simulink model "PGA_MPC_MODEL"  (R2024b)
settings: Solver=ode4  StartTime=0.0  StopTime=180  FixedStep=0.0005  RelTol=1e-3
values from neighbouring files (symbols this model uses):
  Road_Curvature_Map = [Global_S, Global_K]    [Road_Condition_Info.m]
  Road_Mu_Map = [Global_S, Global_Mu]    [Road_Condition_Info.m]
  Target_Speed_Map = [Global_S, Global_Vx]    [Road_Condition_Info.m]
undefined symbols (not defined in the file or in its folder): MotorData, Sim_Mu_Set, Sim_Vx_Set
libraries: Solver_SF x1
(part 1 of 3)
settings Model: Creator=zlm22  LastModifiedBy=zlm22
settings SolverCC: InsertRTBMode=Always
settings RTWCC: BuildConfiguration=Faster Runs

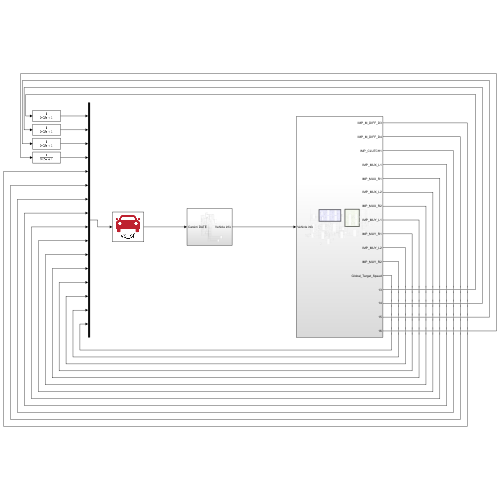
[thumbnail: Simulink's stored preview of the top-level diagram]
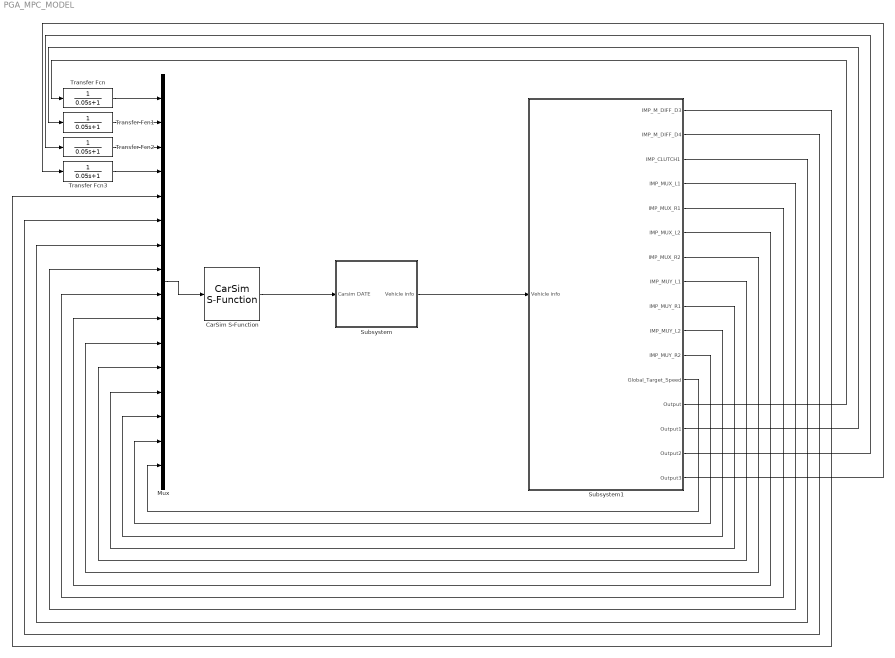
== system PGA_MPC_MODEL ==
  CarSim S-Function : Solver_SF/CarSim S-Function  Priority=1  SIMFILE=simfile.sim  Run_RTs=off  vs_state_ind=Run  StopMode_ind=Vehicle Model
  Mux : Mux  Inputs=16
  Subsystem : Subsystem
  Subsystem1 : Subsystem
  Transfer Fcn{,1..3} (4 alike) : TransferFcn  Denominator=[0.05 1]
  wires:
  Transfer Fcn/1 -> Mux/1
  Transfer Fcn1/1 -> Mux/2
  Transfer Fcn2/1 -> Mux/3
  Transfer Fcn3/1 -> Mux/4
  Subsystem/1(Vehicle info) -> Subsystem1/1(Vehicle info)
  Subsystem1/1(IMP_M_DIFF_D3) -> Mux/5
  Subsystem1/2(IMP_M_DIFF_D4) -> Mux/6
  Subsystem1/3(IMP_CLUTCH1) -> Mux/7
  Subsystem1/4(IMP_MUX_L1) -> Mux/8
  Subsystem1/5(IMP_MUX_R1) -> Mux/9
  Subsystem1/6(IMP_MUX_L2) -> Mux/10
  Subsystem1/7(IMP_MUX_R2) -> Mux/11
  Subsystem1/8(IMP_MUY_L1) -> Mux/12
  Subsystem1/9(IMP_MUY_R1) -> Mux/13
  Subsystem1/10(IMP_MUY_L2) -> Mux/14
  Subsystem1/11(IMP_MUY_R2) -> Mux/15
  Subsystem1/12(Global_Target_Speed) -> Mux/16
  Subsystem1/13(Output) -> Transfer Fcn/1
  Subsystem1/14(Output1) -> Transfer Fcn1/1
  Subsystem1/15(Output2) -> Transfer Fcn2/1
  Subsystem1/16(Output3) -> Transfer Fcn3/1
  Mux/1 -> CarSim S-Function/1
  CarSim S-Function/1 -> Subsystem/1(Carsim DATE)

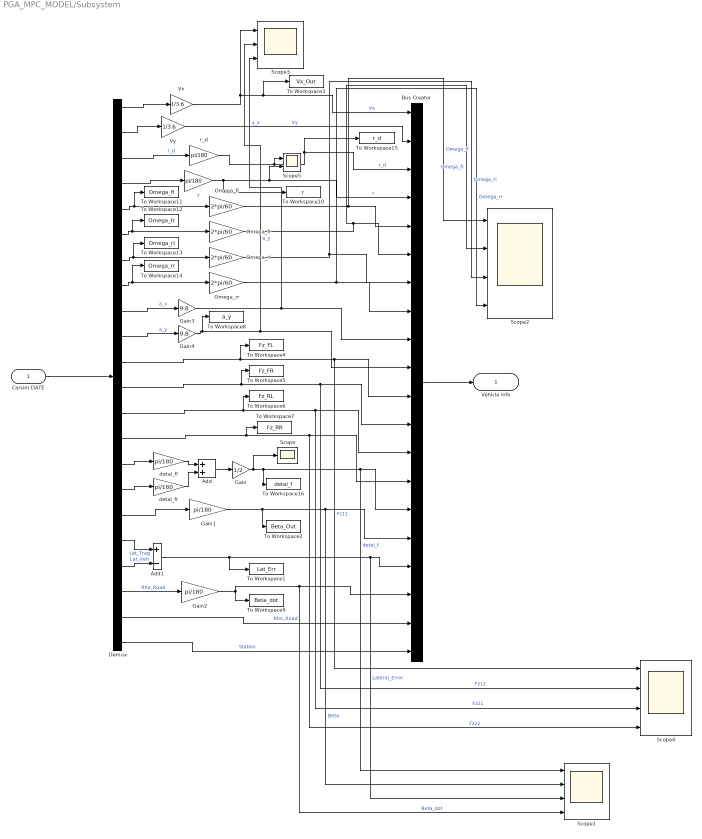
== system PGA_MPC_MODEL/Subsystem ==
  Carsim DATE : Inport
  Add : Sum
  Add1 : Sum  Inputs=+-
  Bus Creator : BusCreator  Inputs=20
  Demux : Demux  Outputs=22
  Gain : Gain  Gain=1/2
  Gain1 : Gain  Gain=pi/180
  Gain2 : Gain  Gain=pi/180
  Gain3 : Gain  Gain=9.8
  Gain4 : Gain  Gain=9.8
  Omega_fl : Gain  Gain=2*pi/60
  Omega_fr : Gain  Gain=2*pi/60
  Omega_rl : Gain  Gain=2*pi/60
  Omega_rr : Gain  Gain=2*pi/60
  Scope : Scope
  Scope1 : Scope  NumInputPorts=4
  Scope2 : Scope  NumInputPorts=4
  Scope3 : Scope  NumInputPorts=3
  Scope4 : Scope  NumInputPorts=4
  Scope5 : Scope  NumInputPorts=2
  To Workspace1 : ToWorkspace  VariableName=Lat_Err  SampleTime=-1
  To Workspace10 : ToWorkspace  VariableName=r  SampleTime=-1
  To Workspace11 : ToWorkspace  VariableName=Omega_fl  SampleTime=-1
  To Workspace12 : ToWorkspace  VariableName=Omega_fr  SampleTime=-1
  To Workspace13 : ToWorkspace  VariableName=Omega_rl  SampleTime=-1
  To Workspace14 : ToWorkspace  VariableName=Omega_rr  SampleTime=-1
  To Workspace15 : ToWorkspace  VariableName=r_d  SampleTime=-1
  To Workspace16 : ToWorkspace  VariableName=detal_f  SampleTime=-1
  To Workspace2 : ToWorkspace  VariableName=Beta_Out  SampleTime=-1
  To Workspace3 : ToWorkspace  VariableName=Vx_Out  SampleTime=-1
  To Workspace4 : ToWorkspace  VariableName=Fz_FL  SaveFormat=Timeseries  SampleTime=-1
  To Workspace5 : ToWorkspace  VariableName=Fz_FR  SaveFormat=Timeseries  SampleTime=-1
  To Workspace6 : ToWorkspace  VariableName=Fz_RL  SaveFormat=Timeseries  SampleTime=-1
  To Workspace7 : ToWorkspace  VariableName=Fz_RR  SaveFormat=Timeseries  SampleTime=-1
  To Workspace8 : ToWorkspace  VariableName=a_y  SampleTime=-1
  To Workspace9 : ToWorkspace  VariableName=Beta_dot  SampleTime=-1
  Vx : Gain  Gain=1/3.6
  Vy : Gain  Gain=1/3.6
  detal_fl : Gain  Gain=pi/180
  detal_fr : Gain  Gain=pi/180
  r : Gain  Gain=pi/180
  r_d : Gain  Gain=pi/180
  Vehicle info : Outport
  wires:
  Demux/3 -> r_d/1  "r_d"
  Demux/11 -> To Workspace4/1, Scope4/1, Bus Creator/11  "Fz11"
  Demux/8 -> To Workspace14/1, Omega_rr/1
  Vy/1 -> Bus Creator/2  "Vy"
  Demux/7 -> To Workspace13/1, Omega_rl/1
  Demux/14 -> To Workspace7/1, Scope4/4, Bus Creator/14  "Fz22"
  Demux/4 -> r/1
  Demux/5 -> To Workspace11/1, Omega_fl/1
  Demux/13 -> To Workspace6/1, Scope4/3, Bus Creator/13  "Fz21"
  Omega_rl/1 -> Scope2/3, Bus Creator/7  "Omega_rl"
  Demux/12 -> To Workspace5/1, Scope4/2, Bus Creator/12  "Fz12"
  Demux/16 -> detal_fr/1
  Omega_fr/1 -> Scope2/2, Bus Creator/6  "Omega_fr"
  Demux/6 -> To Workspace12/1, Omega_fr/1
  Demux/15 -> detal_fl/1
  Vx/1 -> Scope3/1, To Workspace3/1, Bus Creator/1  "Vx"
  r/1 -> Scope5/2, Bus Creator/4, To Workspace10/1  "r"
  Bus Creator/1 -> Vehicle info/1
  Omega_fl/1 -> Scope2/1, Bus Creator/5  "Omega_fl"
  Omega_rr/1 -> Scope2/4, Bus Creator/8  "Omega_rr"
  Demux/10 -> Gain4/1  "a_y"
  Demux/9 -> Gain3/1  "a_x"
  detal_fr/1 -> Add/2
  detal_fl/1 -> Add/1
  Add/1 -> Gain/1
  Gain/1 -> Scope/1, To Workspace16/1, Scope1/1, Bus Creator/15  "detal_f"
  Demux/1 -> Vx/1
  Demux/2 -> Vy/1
  Demux/17 -> Gain1/1
  Gain1/1 -> To Workspace2/1, Bus Creator/16, Scope1/2  "Beta"
  Gain2/1 -> Scope1/4, Bus Creator/18, To Workspace9/1  "Beta_dot"
  r_d/1 -> To Workspace15/1, Bus Creator/3, Scope5/1  "r_d"
  Carsim DATE/1 -> Demux/1
  Gain4/1 -> To Workspace8/1, Scope3/2, Bus Creator/10  "a_y"
  Gain3/1 -> Scope3/3, Bus Creator/9  "a_x"
  Demux/22 -> Bus Creator/20  "Station"
  Demux/21 -> Bus Creator/19  "Rho_Road"
  Demux/20 -> Gain2/1  "Rho_Road"
  Demux/18 -> Add1/1  "Lat_Trag"
  Demux/19 -> Add1/2  "Lat_Veh"
  Add1/1 -> To Workspace1/1, Scope1/3, Bus Creator/17  "Lateral_Error"

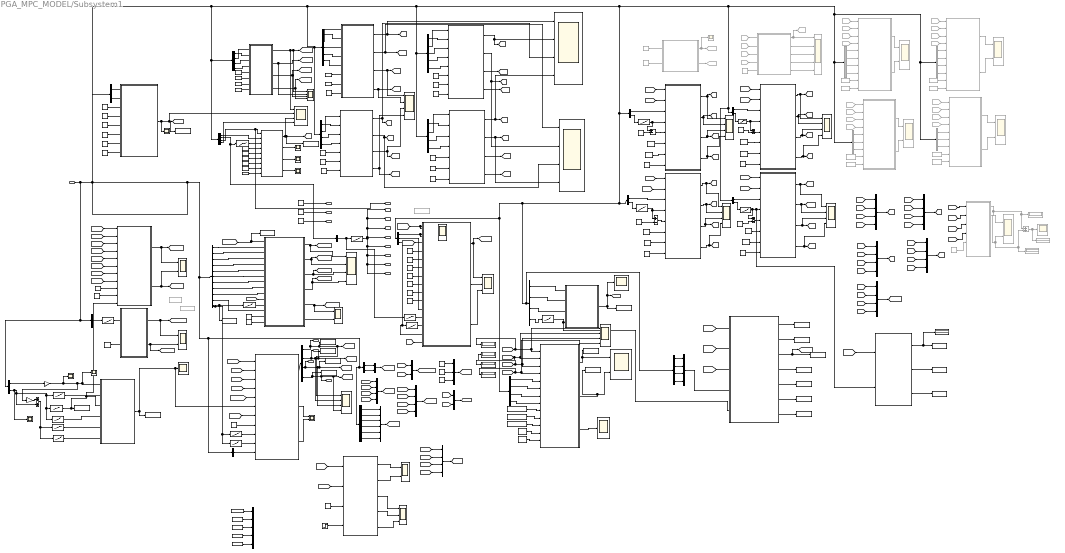
== system PGA_MPC_MODEL/Subsystem1 ==
  note: Subsystem3
  note: 轮胎力
  Vehicle info : Inport
  Add1 : Sum  Commented=on
  Add{2..4,6} (4 alike) : Sum  Inputs=+-
  Add5 : Sum
  Bus Creator : BusCreator  Inputs=6
  Bus Creator1 : BusCreator  Inputs=2
  Bus Selector : BusSelector  OutputSignals=Omega_fl,Omega_fr,Omega_rl,Omega_rr,Fz11,Fz12,Fz21,Fz22,a_y,Lateral_Error,Station
  Bus Selector1 : BusSelector  OutputSignals=Vx,detal_f,Fz11,Fz12,Fz21,Fz22
  Bus Selector10 : BusSelector  OutputSignals=Fz11,Station
  Bus Selector11 : BusSelector  OutputSignals=Fz21,Station
  Bus Selector12 : BusSelector  OutputSignals=Fz12,Station
  Bus Selector13 : BusSelector  OutputSignals=Fz22,Station
  Bus Selector15 : BusSelector  OutputSignals=Vx,Station
  Bus Selector16 : BusSelector  OutputSignals=detal_f
  Bus Selector17 : BusSelector  Commented=on  OutputSignals=Vx,Vy,r_d,detal_f
  Bus Selector18 : BusSelector  OutputSignals=Fz11,Fz12,Fz21,Fz22
  Bus Selector19 : BusSelector  Commented=on  OutputSignals=Vx,Vy,r_d,detal_f
  Bus Selector2 : BusSelector  OutputSignals=Beta,r_d
  Bus Selector20 : BusSelector  Commented=on  OutputSignals=Vx,Vy,r_d
  Bus Selector21 : BusSelector  Commented=on  OutputSignals=Vx,Vy,r_d
  Bus Selector22 : BusSelector  OutputSignals=Station
  Bus Selector23 : BusSelector  OutputSignals=detal_f,Station,Vx,r_d
  Bus Selector24 : BusSelector  OutputSignals=Station
  Bus Selector25 : BusSelector  OutputSignals=Omega_fl,Omega_fr,Omega_rl,Omega_rr
  Bus Selector26 : BusSelector  OutputSignals=Vx,detal_f,Beta
  Bus Selector27 : BusSelector  OutputSignals=Vx,Beta,Beta_dot,Station
  Bus Selector3 : BusSelector  OutputSignals=Vx,detal_f
  Bus Selector5 : BusSelector  OutputSignals=Vy,Vx,r_d,Omega_fl,detal_f
  Bus Selector6 : BusSelector  OutputSignals=Vy,Vx,r_d,detal_f
  Bus Selector7 : BusSelector  OutputSignals=Vy,Vx,r_d,Omega_fr,detal_f
  Bus Selector8 : BusSelector  OutputSignals=Vy,Vx,r_d,Omega_rl
  Bus Selector9 : BusSelector  OutputSignals=Vy,Vx,r_d,Omega_rr
  Constant{1,7,18,21,48} (5 alike) : Constant  Value=1.152
  Constant{2,8,10,13,49} (5 alike) : Constant  Value=1.528
  Constant{9,11,14,16..17,19} (6 alike) : Constant  Value=1.565
  Constant{12,15,20,22,54} (5 alike) : Constant  Value=0.347
  Constant{23..25,60,82} (5 alike) : Constant  Value=0
  Constant{26,73,81,84,91} (5 alike) : Constant  Value=0.05
  Constant27 : Constant  Commented=on  Value=3
  Constant28 : Constant  Commented=on  Value=0.001
  Constant{29,32,35,38} (4 alike) : Constant  Value=0.6
  Constant{3,31,37,50,79} (5 alike) : Constant  Value=63833
  Constant30 : Constant  Commented=on  Value=1.152
  Constant33 : Constant  Value=44230
  Constant{4,34,40,51,88} (5 alike) : Constant  Value=48729
  Constant36 : Constant  Value=57917
  Constant39 : Constant  Value=44230
  Constant41 : Constant  Commented=on  Value=0.347
  Constant{6,42,59,61,86} (5 alike) : Constant  Value=0.01
  Constant43 : Constant  Value=800
  Constant44 : Constant  Commented=on  Value=Sim_Mu_Set
  Constant45 : Constant  Value=MotorData.Speed_Axis
  Constant47 : Constant  Value=1810
  Constant5 : Constant  Value=1810
  Constant52 : Constant  Value=9.81
  Constant53 : Constant  Value=MotorData.Torque_Axis
  Constant55 : Constant  Value=1810
  Constant56 : Constant  Value=9.81
  Constant57 : Constant  Value=12
  Constant58 : Constant  Value=0.3
  Constant66 : Constant  Commented=on  Value=Sim_Vx_Set
  Constant68 : Constant  Commented=on  Value=Sim_Vx_Set
  Constant75 : Constant  Value=8000
  Constant76 : Constant  Value=12000
  Constant77 : Constant  Value=MotorData.Eff_Map
  Constant{78,92,94,96} (4 alike) : Constant  Commented=on  Value=1.565
  Constant80 : Constant  Value=0.005
  Constant83 : Constant  Value=18000
  Constant85 : Constant  Value=20000
  Constant87 : Constant  Value=15000  VectorParams1D=off
  Constant89 : Constant  Value=57917
  Constant90 : Constant  Commented=on  Value=1.152
  Constant93 : Constant  Commented=on  Value=1.528
  Constant95 : Constant  Commented=on  Value=1.528
  Constant97 : Constant  Commented=on  Value=0.01
  Demux : Demux
  Display{,1..3,8} (5 alike) : Display
  Display4 : Display  Commented=on
  Display5 : Display  Commented=on
  Display6 : Display  Commented=on
  From : From  Commented=on  GotoTag=Fx_fl
  From36 : From  Commented=on  GotoTag=Fx_fr
  From40 : From  Commented=on  GotoTag=Sx_fr
  From41 : From  Commented=on  GotoTag=Sy_fr
  From42 : From  Commented=on  GotoTag=Fy_rl
  From43 : From  Commented=on  GotoTag=Sx_rl
  From44 : From  Commented=on  GotoTag=Sy_rl
  From45 : From  Commented=on  GotoTag=Fx_rl
  From46 : From  Commented=on  GotoTag=Fy_rr
  From47 : From  Commented=on  GotoTag=Sx_rr
  From48 : From  Commented=on  GotoTag=Sy_rr
  From49 : From  Commented=on  GotoTag=Fx_rr
  From5 : From  Commented=on  GotoTag=Fy_fl
  From6 : From  Commented=on  GotoTag=Sx_fl
  From68 : From  Commented=on  GotoTag=Fx_fl
  From69 : From  Commented=on  GotoTag=Fx_fr
  From7 : From  Commented=on  GotoTag=Sy_fl
  From70 : From  Commented=on  GotoTag=Fx_rl
  From71 : From  Commented=on  GotoTag=Fx_rr
  From8 : From  Commented=on  GotoTag=Fx_fr
  Gain : Gain  Gain=3.6
  Gain2 : Gain  Gain=1.2
  Goto29 : Goto  Commented=on  GotoTag=mu_y
  Goto5 : Goto  Commented=on  GotoTag=mu_x
  MATLAB Function : MATLAB Function  TreatAsAtomicUnit=on  SystemSampleTime=0.01
  MATLAB Function1 : MATLAB Function  TreatAsAtomicUnit=on
  MATLAB Function10 : MATLAB Function  TreatAsAtomicUnit=on
  MATLAB Function12 : MATLAB Function  TreatAsAtomicUnit=on
  MATLAB Function14 : MATLAB Function  TreatAsAtomicUnit=on
  MATLAB Function15 : MATLAB Function  TreatAsAtomicUnit=on  SystemSampleTime=0.01
  MATLAB Function16 : MATLAB Function  Commented=on  TreatAsAtomicUnit=on
  MATLAB Function17 : MATLAB Function  TreatAsAtomicUnit=on
  MATLAB Function18 : MATLAB Function  TreatAsAtomicUnit=on
  MATLAB Function19 : MATLAB Function  TreatAsAtomicUnit=on  SystemSampleTime=0.01
  MATLAB Function2 : MATLAB Function  TreatAsAtomicUnit=on  SystemSampleTime=0.01
  MATLAB Function20 : MATLAB Function  Commented=on  TreatAsAtomicUnit=on
  MATLAB Function21 : MATLAB Function  Commented=on  TreatAsAtomicUnit=on  SystemSampleTime=0.01
  MATLAB Function22 : MATLAB Function  Commented=on  TreatAsAtomicUnit=on
  MATLAB Function23 : MATLAB Function  TreatAsAtomicUnit=on  SystemSampleTime=0.01
  MATLAB Function24 : MATLAB Function  Commented=on  TreatAsAtomicUnit=on
  MATLAB Function25 : MATLAB Function  Commented=on  TreatAsAtomicUnit=on
  MATLAB Function26 : MATLAB Function  TreatAsAtomicUnit=on
  MATLAB Function27 : MATLAB Function  TreatAsAtomicUnit=on
  MATLAB Function3 : MATLAB Function  TreatAsAtomicUnit=on  SystemSampleTime=0.01
  MATLAB Function4 : MATLAB Function  TreatAsAtomicUnit=on
  MATLAB Function5 : MATLAB Function  TreatAsAtomicUnit=on
  MATLAB Function6 : MATLAB Function  TreatAsAtomicUnit=on
  MATLAB Function7 : MATLAB Function  TreatAsAtomicUnit=on
  MATLAB Function8 : MATLAB Function  TreatAsAtomicUnit=on
  MATLAB Function9 : MATLAB Function  TreatAsAtomicUnit=on
  MU : Lookup_n-D  NumberOfTableDimensions=1  BreakpointsForDimension1=Road_Mu_Map(:, 1)  Table=Road_Mu_Map(:, 2)  InternalRulePriority=Speed  RndMeth=Simplest
  Mu{2..9,12..14} (11 alike) : Lookup_n-D  NumberOfTableDimensions=1  BreakpointsForDimension1=Road_Mu_Map(:, 1)  Table=Road_Mu_Map(:, 2)  InternalRulePriority=Speed  RndMeth=Simplest
  Mux : Mux  Inputs=2
  Mux{1,3,5..10,12} (9 alike) : Mux
  Mux13 : Mux  Inputs=5
  Mux2 : Mux  Inputs=2
  Mux4 : Mux  Inputs=3
  Radius{1..4} (4 alike) : Lookup_n-D  NumberOfTableDimensions=1  BreakpointsForDimension1=Road_Curvature_Map(:, 1)  Table=Road_Curvature_Map(:, 2)  InternalRulePriority=Speed  RndMeth=Simplest
  SI : Scope
  Scope{,1..2,5,27,37,45} (7 alike) : Scope  NumInputPorts=2
  Scope{10..14} (5 alike) : Scope  Commented=on  NumInputPorts=2
  Scope{3..4,6,9,15..18,20,28,30,48} (12 alike) : Scope  NumInputPorts=4
  Scope{8,19,21..22,32..34,44,49} (9 alike) : Scope
  Scope23 : Scope  Commented=on
  Scope24 : Scope  Commented=on  NumInputPorts=5
  Scope29 : Scope  NumInputPorts=3
  Scope47 : Scope  Commented=on
  Scope7 : Scope  NumInputPorts=3
  Step : Step  Time=0.01  Before=1  After=0  SampleTime=0.01
  T_max : Constant  Value=800
  T_min : Constant  Value=-200
  To Workspace : ToWorkspace  VariableName=SI_Out  SaveFormat=Timeseries  SampleTime=-1
  To Workspace10 : ToWorkspace  VariableName=R_ref  SampleTime=-1
  To Workspace12 : ToWorkspace  VariableName=beta_ref  SampleTime=-1
  To Workspace13 : ToWorkspace  VariableName=Sim_Station  SampleTime=-1
  To Workspace14 : ToWorkspace  VariableName=Mu  SampleTime=-1
  To Workspace17 : ToWorkspace  VariableName=Sx_abs_vec  SampleTime=-1
  To Workspace18 : ToWorkspace  VariableName=Sx_max  SampleTime=-1
  To Workspace19 : ToWorkspace  VariableName=Sx_rms  SampleTime=-1
  To Workspace2 : ToWorkspace  VariableName=NN_Weights  SampleTime=-1
  To Workspace20 : ToWorkspace  VariableName=Eta_vec  SampleTime=-1
  To Workspace21 : ToWorkspace  VariableName=Eta_max  SampleTime=-1
  To Workspace22 : ToWorkspace  VariableName=Eta_rms  SampleTime=-1
  To Workspace23 : ToWorkspace  VariableName=Slip_Debug_Info  SampleTime=-1
  To Workspace24 : ToWorkspace  VariableName=I_Sx  SampleTime=-1
  To Workspace25 : ToWorkspace  VariableName=I_Sx_norm  SampleTime=-1
  To Workspace26 : ToWorkspace  VariableName=I_Debug  SampleTime=-1
  To Workspace3 : ToWorkspace  VariableName=Total_Power_Out  SampleTime=-1
  To Workspace4 : ToWorkspace  VariableName=Motor_Torque_FL  SampleTime=-1
  To Workspace5 : ToWorkspace  VariableName=Motor_Torque_FR  SampleTime=-1
  To Workspace6 : ToWorkspace  VariableName=Motor_Torque_RL  SampleTime=-1
  To Workspace7 : ToWorkspace  VariableName=Motor_Torque_RR  SampleTime=-1
  To Workspace8 : ToWorkspace  VariableName=E_total_kWh  SampleTime=-1
  To Workspace9 : ToWorkspace  VariableName=P_total_kW  SampleTime=-1
  Vx1 : Lookup_n-D  NumberOfTableDimensions=1  BreakpointsForDimension1=Target_Speed_Map(:, 1)  Table=Target_Speed_Map(:, 2)  InternalRulePriority=Speed  RndMeth=Simplest
  Vx2 : Lookup_n-D  NumberOfTableDimensions=1  BreakpointsForDimension1=Target_Speed_Map(:, 1)  Table=Target_Speed_Map(:, 2)  InternalRulePriority=Speed  RndMeth=Simplest
  delta_T_max : Constant  Value=600
  unitire轮胎力 : MATLAB Function  TreatAsAtomicUnit=on
  侧偏角计算 : MATLAB Function  TreatAsAtomicUnit=on
  总需求扭矩 : Goto  Commented=on  GotoTag=Td
  横纵向附着系数 : MATLAB Function  Commented=on  TreatAsAtomicUnit=on
  IMP_M_DIFF_D3 : Outport
  IMP_M_DIFF_D4 : Outport  Port=2
  IMP_CLUTCH1 : Outport  Port=3
  IMP_MUX_L1 : Outport  Port=4
  IMP_MUX_R1 : Outport  Port=5
  IMP_MUX_L2 : Outport  Port=6
  IMP_MUX_R2 : Outport  Port=7
  IMP_MUY_L1 : Outport  Port=8
  IMP_MUY_R1 : Outport  Port=9
  IMP_MUY_L2 : Outport  Port=10
  IMP_MUY_R2 : Outport  Port=11
  Global_Target_Speed : Outport  Port=12
  Output : Outport  Port=13
  Output1 : Outport  Port=14
  Output2 : Outport  Port=15
  Output3 : Outport  Port=16
  wires:
  MATLAB Function5/1(Sx_fr) -> [Sx_fr], Scope9/2
  Bus Selector7/1 -> MATLAB Function5/2(Vy)  "<Vy>"
  Constant13/1 -> MATLAB Function7/5(lr)
  Constant21/1 -> MATLAB Function5/6(lf)
  MATLAB Function8/3(Fbar_x_rl) -> Scope17/3, [Fsx_rl]
  MATLAB Function6/1(Sx_rl) -> [Sx_rl], Scope9/3
  Constant14/1 -> MATLAB Function7/6(twr)
  MATLAB Function7/1(Sx_rr) -> [Sx_rr], Scope9/4
  Constant1/1 -> MATLAB Function4/3(lf)
  Bus Selector11/1 -> MATLAB Function8/3(Fz_rl)  "<Fz21>"
  MATLAB Function9/2(Fy_fr) -> Scope15/2, [Fy_fr]
  Bus Selector6/4 -> 侧偏角计算/4(delta_f_rad)  "<detal_f>"
  MATLAB Function5/2(Sy_fr) -> [Sy_fr], Scope28/2
  Constant47/1 -> MATLAB Function17/4(m)
  Bus Selector5/5 -> unitire轮胎力/5(delta_f)  "<detal_f>"
  [Sx_fr] -> MATLAB Function9/1(Sx_fr)
  Constant52/1 -> MATLAB Function17/9(g)
  MATLAB Function17/1(r_d) -> [r_ref], To Workspace10/1, Scope30/3  "r_ref"
  Constant15/1 -> MATLAB Function7/7(Re)
  MATLAB Function9/1(Fx_fr) -> Scope15/1, [Fx_fr]
  MATLAB Function10/1(Fx_rr) -> Scope18/1, [Fx_rr]
  MATLAB Function1/1(Fx_fl) -> [Fx_fl], Scope48/1
  MATLAB Function7/2(Sy_rr) -> Scope28/4, [Sy_rr]
  Constant2/1 -> MATLAB Function4/4(lr)
  MATLAB Function20/1(Td) -> Scope24/1, 总需求扭矩/1
  Constant38/1 -> MATLAB Function10/8(E)
  [Sy_fr] -> MATLAB Function9/2(Sy_fr)
  Constant9/1 -> 侧偏角计算/7(twf)
  Bus Selector10/1 -> MATLAB Function1/3(Fz_fl)  "<Fz11>"
  Bus Selector7/4 -> MATLAB Function5/4(omega_fr)  "<Omega_fr>"
  Constant4/1 -> MATLAB Function4/6(Kyr)
  Constant5/1 -> MATLAB Function4/7(m)
  Constant8/1 -> 侧偏角计算/6(lr)
  Constant27/1 -> 横纵向附着系数/1(road_condition)
  Bus Selector3/2 -> MATLAB Function4/2(delta_f)  "<detal_f>"
  Bus Selector3/1 -> MATLAB Function4/1(Vx)  "<Vx>"
  Constant6/1 -> MATLAB Function4/8(dt)
  Constant17/1 -> MATLAB Function5/7(twf)
  MATLAB Function4/1(beta_ref) -> Scope44/1, To Workspace12/1, [beta_ref], Scope30/2  "beta_ref"
  MATLAB Function1/3(Fbar_x_fl) -> Scope48/3, [Fsx_fl]
  Constant48/1 -> MATLAB Function17/5(lf)
  Constant3/1 -> MATLAB Function4/5(Kyf)
  MATLAB Function1/4(Fbar_y_fl) -> Scope48/4, [Fsy_fl]
  Constant29/1 -> MATLAB Function1/8(E)
  From68/1 -> MATLAB Function20/1(Fx_fl)
  Bus Selector8/4 -> MATLAB Function6/4(omega_rl)  "<Omega_rl>"
  MATLAB Function6/2(Sy_rl) -> Scope28/3, [Sy_rl]
  From71/1 -> MATLAB Function20/4(Fx_rr)
  Constant50/1 -> MATLAB Function17/7(Kf0)
  Bus Selector5/4 -> unitire轮胎力/4(omega_fl)  "<Omega_fl>"
  Bus Selector6/1 -> 侧偏角计算/2(Vy)  "<Vy>"
  Constant49/1 -> MATLAB Function17/6(lr)
  MATLAB Function8/4(Fbar_y_rl) -> Scope17/4, [Fsy_rl]
  MATLAB Function9/4(Fbar_y_fr) -> Scope15/4, [Fsy_fr]
  Constant51/1 -> MATLAB Function17/8(Kr0)
  MATLAB Function17/4(r_limit) -> Scope34/1
  MATLAB Function17/2(K_s) -> Scope32/1
  MATLAB Function17/3(r_ideal) -> Scope33/1
  Constant22/1 -> MATLAB Function5/8(Re)
  横纵向附着系数/1(mu_x) -> Scope47/1, Goto5/1
  Bus Selector12/1 -> MATLAB Function9/3(Fz_fr)  "<Fz12>"
  [Sx_fl] -> MATLAB Function1/1(Sx_fl)
  Bus Selector9/4 -> MATLAB Function7/4(omega_rr)  "<Omega_rr>"
  unitire轮胎力/1(Sx_fl) -> Scope9/1, [Sx_fl]
  From69/1 -> MATLAB Function20/2(Fx_fr)
  From70/1 -> MATLAB Function20/3(Fx_rl)
  Constant10/1 -> MATLAB Function6/5(lr)
  [Sy_rr] -> MATLAB Function10/2(Sy_rr)
  Constant41/1 -> MATLAB Function20/5(r_e)
  Constant35/1 -> MATLAB Function9/8(E)
  [Sy_rl] -> MATLAB Function8/2(Sy_rl)
  Constant7/1 -> 侧偏角计算/5(lf)
  MATLAB Function9/3(Fbar_x_fr) -> Scope15/3, [Fsx_fr]
  Bus Selector13/1 -> MATLAB Function10/3(Fz_rr)  "<Fz22>"
  MATLAB Function1/2(Fy_fl) -> [Fy_fl], Scope48/2
  MATLAB Function10/4(Fbar_y_rr) -> Scope18/4, [Fsy_rr]
  MATLAB Function10/2(Fy_rr) -> Scope18/2, [Fy_rr]
  MATLAB Function10/3(Fbar_x_rr) -> Scope18/3, [Fsx_rr]
  Mu5/1 -> Add6/1, MATLAB Function1/4(mu_x)
  [Sx_rr] -> MATLAB Function10/1(Sx_rr)
  Constant32/1 -> MATLAB Function8/8(E)
  MATLAB Function8/1(Fx_rl) -> Scope17/1, [Fx_rl]
  MATLAB Function8/2(Fy_rl) -> Scope17/2, [Fy_rl]
  [Sy_fl] -> MATLAB Function1/2(Sy_fl)
  Constant19/1 -> unitire轮胎力/7(twf)
  [Sx_rl] -> MATLAB Function8/1(Sx_rl)
  横纵向附着系数/2(mu_y) -> Goto29/1
  Constant28/1 -> 横纵向附着系数/2(slip_ratio)
  Bus Selector9/1 -> MATLAB Function7/2(Vy)  "<Vy>"
  Constant18/1 -> unitire轮胎力/6(lf)
  unitire轮胎力/2(Sy_fl) -> Scope28/1, [Sy_fl]
  Constant16/1 -> 侧偏角计算/8(twr)
  Constant11/1 -> MATLAB Function6/6(twr)
  Bus Selector8/1 -> MATLAB Function6/2(Vy)  "<Vy>"
  Constant20/1 -> unitire轮胎力/8(Re)
  Bus Selector5/1 -> unitire轮胎力/2(Vy)  "<Vy>"
  Vehicle info/1 -> Bus Selector15/1, Bus Selector24/1, Bus Selector/1, Bus Selector1/1, Bus Selector2/1, Bus Selector16/1, Bus Selector23/1, Bus Selector6/1, Bus Selector9/1, Bus Selector7/1, Bus Selector10/1, Bus Selector18/1, Bus Selector27/1, Bus Selector25/1, Bus Selector26/1, Bus Selector11/1, Bus Selector21/1, Bus Selector19/1, Bus Selector20/1, Bus Selector17/1, Bus Selector13/1, Bus Selector12/1, Bus Selector8/1, Bus Selector5/1, Bus Selector3/1
  MATLAB Function20/5(T_rr) -> Scope24/5
  MATLAB Function20/4(T_rl) -> Scope24/4
  MATLAB Function20/3(T_fr) -> Scope24/3
  MATLAB Function20/2(T_fl) -> Scope24/2
  [T_ZY_RR] -> Display3/1, Scope6/4, MATLAB Function2/4(T_rr)
  [T_ZY_RL] -> Display2/1, Scope6/3, MATLAB Function2/3(T_rl)
  [T_ZY_FL] -> Display/1, Scope6/1, MATLAB Function2/1(T_fl)
  [T_ZY_FR] -> Display1/1, Scope6/2, MATLAB Function2/2(T_fr)
  Bus Selector25/1 -> MATLAB Function2/5(w_fl)  "<Omega_fl>"
  Bus Selector25/2 -> MATLAB Function2/6(w_fr)  "<Omega_fr>"
  Bus Selector25/3 -> MATLAB Function2/7(w_rl)  "<Omega_rl>"
  MATLAB Function2/3(P_avg_kW) -> Scope49/1
  Constant55/1 -> MATLAB Function15/4(m)
  Constant56/1 -> MATLAB Function15/5(g)
  MATLAB Function15/1(T_total) -> [T_total], Scope7/1
  MATLAB Function18/1(Vx_safe_cmd) -> Scope45/1, [Vx_safe_cmd]
  MATLAB Function18/2(Ax_cmd_final) -> Scope45/2, [Ax_cmd_final]
  [Vx_safe_cmd] -> Scope37/1, MATLAB Function15/1(Vx_cmd)
  [Ax_cmd_final] -> MATLAB Function15/3(Ax_cmd)
  MATLAB Function2/2(E_total_kWh) -> To Workspace8/1, Scope2/2
  MATLAB Function2/1(P_total_kW) -> To Workspace9/1, Scope2/1
  Constant73/1 -> MATLAB Function18/2(dt)
  Bus Selector27/3 -> MATLAB Function19/3(Beta_dot)  "<Beta_dot>"
  MATLAB Function19/1(SI_Out) -> SI/1, [SI], To Workspace/1  "SI_Out"
  [Fy_fl] -> MATLAB Function23/1(Fy_fl)
  [Fy_fr] -> MATLAB Function23/2(Fy_fr)
  [Fy_rl] -> MATLAB Function23/3(Fy_rl)
  [Fy_rr] -> MATLAB Function23/4(Fy_rr)
  [alpha_fl] -> MATLAB Function23/5(Alpha_fl)
  [alpha_fr] -> MATLAB Function23/6(Alpha_fr)
  [alpha_rl] -> MATLAB Function23/7(Alpha_rl)
  [alpha_rr] -> MATLAB Function23/8(Alpha_rr)
  Constant88/1 -> MATLAB Function23/10(Cr0)
  Constant79/1 -> MATLAB Function23/9(Cf0)
  MATLAB Function23/1(Cf_eq) -> Scope5/1, [Cf_eq]
  MATLAB Function23/2(Cr_eq) -> Scope5/2, [Cr_eq]
  Constant23/1 -> IMP_M_DIFF_D3/1
  Constant24/1 -> IMP_M_DIFF_D4/1
  Constant25/1 -> IMP_CLUTCH1/1
  Mu3/1 -> IMP_MUX_R2/1, IMP_MUX_L2/1, IMP_MUX_R1/1, IMP_MUX_L1/1, IMP_MUY_L1/1, IMP_MUY_R1/1, IMP_MUY_L2/1, IMP_MUY_R2/1
  Constant81/1 -> Add2/2
  Constant84/1 -> Add3/2
  Add4/1 -> MATLAB Function8/5(mu_y)
  Mu7/1 -> MATLAB Function8/4(mu_x), Add4/1
  Constant91/1 -> Add4/2
  [T_total] -> To Workspace3/1, MATLAB Function3/1(T_total_req)
  Bus Selector/8 -> MATLAB Function3/9(Fz_rr)  "<Fz22>"
  Bus Selector/7 -> MATLAB Function3/8(Fz_rl)  "<Fz21>"
  Bus Selector/6 -> MATLAB Function3/7(Fz_fr)  "<Fz12>"
  Bus Selector/5 -> MATLAB Function3/6(Fz_fl)  "<Fz11>"
  Bus Selector/4 -> MATLAB Function3/5(w_rr)  "<Omega_rr>"
  Bus Selector/3 -> MATLAB Function3/4(w_rl)  "<Omega_rl>"
  Bus Selector/2 -> MATLAB Function3/3(w_fr)  "<Omega_fr>"
  Bus Selector/1 -> MATLAB Function3/2(w_fl)  "<Omega_fl>"
  Constant43/1 -> MATLAB Function3/14(T_motor_max)
  MATLAB Function3/5(Mode_Out) -> Scope/1, [Mode_Signal]
  MATLAB Function3/1(T_ref_fl) -> [T_ref_fl], Scope4/1
  MATLAB Function3/2(T_ref_fr) -> Scope4/2, [T_ref_fr]
  MATLAB Function3/3(T_ref_rl) -> [T_ref_rl], Scope4/3
  MATLAB Function3/4(T_ref_rr) -> [T_ref_rr], Scope4/4
  Constant42/1 -> MATLAB Function3/15(dt)
  [beta_ref] -> Mux/1
  [r_ref] -> Mux/2
  [T_ref_fl] -> Mux1/1
  [T_ref_fr] -> Mux1/2
  [T_ref_rl] -> Mux1/3
  [T_ref_rr] -> Mux1/4
  Mux1/1 -> [T_ref_upper]
  [Cf_eq] -> Mux2/1
  [Cr_eq] -> Mux2/2
  Mux2/1 -> [Stiffness_Input]
  Bus Selector1/3 -> Bus Creator/3  "<Fz11>"
  Bus Selector1/4 -> Bus Creator/4  "<Fz12>"
  Bus Selector1/5 -> Bus Creator/5  "<Fz21>"
  Bus Selector1/6 -> Bus Creator/6  "<Fz22>"
  Bus Creator/1 -> [Vehicle_State]
  Bus Selector2/1 -> Bus Creator1/1  "<Beta>"
  Bus Selector2/2 -> Bus Creator1/2  "<r_d>"
  Bus Creator1/1 -> [x_curr]
  T_min/1 -> Mux4/1
  T_max/1 -> Mux4/2
  delta_T_max/1 -> Mux4/3
  Mux4/1 -> [Constraints]
  [x_curr] -> MATLAB Function/1(x_curr)
  [x_ref] -> MATLAB Function/2(x_ref)
  [T_ref_upper] -> MATLAB Function/3(T_ref_upper_in)
  [Vehicle_State] -> MATLAB Function/4(Vehicle_State)
  [Stiffness_Input] -> MATLAB Function/5(Stiffness_Input)
  [Constraints] -> MATLAB Function/7(Constraints)
  MATLAB Function/2(Solver_Status) -> Scope1/1
  MATLAB Function/3(Debug_Info) -> Scope1/2
  MATLAB Function/1(T_final_opt) -> Demux/1
  Demux/1 -> Output/1, To Workspace4/1, [T_ZY_FL], Scope3/1  "F11"
  Demux/2 -> Output1/1, To Workspace5/1, [T_ZY_FR], Scope3/2  "F12"
  Demux/3 -> Output2/1, To Workspace6/1, [T_ZY_RL], Scope3/3  "F21"
  Demux/4 -> To Workspace7/1, Output3/1, Scope3/4, [T_ZY_RR]  "F22"
  Constant54/1 -> MATLAB Function15/6(r_e)
  Constant60/1 -> MATLAB Function15/10(is_reset)
  Constant58/1 -> MATLAB Function15/8(Ki)
  Constant57/1 -> MATLAB Function15/7(Kp)
  Constant59/1 -> MATLAB Function15/9(dt)
  MATLAB Function15/2(T_ff) -> Scope7/2
  MATLAB Function15/3(T_fb) -> Scope7/3
  [alpha_fl] -> Mux5/1
  [alpha_fr] -> Mux5/2
  [alpha_rl] -> Mux5/3
  [alpha_rr] -> Mux5/4
  Mux5/1 -> [SlipAngles_in]
  Bus Selector/9 -> MATLAB Function3/10(Ay_in)  "<a_y>"
  [SI] -> MATLAB Function3/11(SI_in)
  Mu2/1 -> MATLAB Function3/12(Mu_in)
  Mu4/1 -> MATLAB Function17/3(mu)
  Mu9/1 -> MATLAB Function26/5(Mu_in), MATLAB Function19/4(mu)
  Bus Selector25/4 -> MATLAB Function2/8(w_rr)  "<Omega_rr>"
  Constant45/1 -> MATLAB Function2/9(Map_Spd)
  Constant53/1 -> MATLAB Function2/10(Map_Trq)
  Constant77/1 -> MATLAB Function2/11(Map_Eff)
  Constant80/1 -> MATLAB Function2/12(dt)
  Constant82/1 -> MATLAB Function2/13(is_reset)
  Constant86/1 -> MATLAB Function/8(dt_in)
  Bus Selector/10 -> MATLAB Function3/13(Lat_Error_in)  "<Lateral_Error>"
  侧偏角计算/1(alpha_fl) -> Scope20/1, [alpha_fl], Scope30/1  "alpha_fl"
  侧偏角计算/2(alpha_fr) -> [alpha_fr], Scope20/2  "alpha_fr"
  侧偏角计算/3(alpha_rl) -> [alpha_rl], Scope20/3  "alpha_rl"
  侧偏角计算/4(alpha_rr) -> [alpha_rr], Scope20/4  "alpha_rr"
  Constant12/1 -> MATLAB Function6/7(Re)
  Bus Selector7/5 -> MATLAB Function5/5(delta_f)  "<detal_f>"
  Bus Selector5/3 -> unitire轮胎力/3(r)  "<r_d>"
  Bus Selector7/3 -> MATLAB Function5/3(r)  "<r_d>"
  Bus Selector8/3 -> MATLAB Function6/3(r)  "<r_d>"
  Bus Selector9/3 -> MATLAB Function7/3(r)  "<r_d>"
  Constant26/1 -> Add6/2
  Add6/1 -> MATLAB Function1/5(mu_y)
  Constant89/1 -> MATLAB Function1/6(Kx)
  Constant31/1 -> MATLAB Function1/7(Ky)
  Mu6/1 -> MATLAB Function9/4(mu_x), Add2/1
  Add2/1 -> MATLAB Function9/5(mu_y)
  Constant36/1 -> MATLAB Function9/6(Kx)
  Constant37/1 -> MATLAB Function9/7(Ky)
  Constant33/1 -> MATLAB Function8/6(Kx)
  Constant34/1 -> MATLAB Function8/7(Ky)
  Add3/1 -> MATLAB Function10/5(mu_y)
  Mu8/1 -> Add3/1, MATLAB Function27/2(Station_m), MATLAB Function10/4(mu_x)
  Constant39/1 -> MATLAB Function10/6(Kx)
  Constant40/1 -> MATLAB Function10/7(Ky)
  unitire轮胎力/3(Vsx_fl) -> Scope16/1, [Vsx_fl]
  unitire轮胎力/4(Vsy_fl) -> Scope16/2, [Vsy_fl]
  MATLAB Function6/3(Vsx_rl) -> [Vsx_rl], Scope16/3
  MATLAB Function6/4(Vsy_rl) -> [Vsy_rl], Scope16/4
  MATLAB Function7/3(Vsx_rr) -> [Vsx_rr]
  MATLAB Function7/4(Vsy_rr) -> [Vsy_rr]
  Bus Selector17/4 -> MATLAB Function16/8(delta_f)  "<detal_f>"
  Bus Selector17/3 -> MATLAB Function16/7(r)  "<r_d>"
  Bus Selector17/2 -> MATLAB Function16/6(Vy)  "<Vy>"
  Bus Selector17/1 -> MATLAB Function16/5(Vx)  "<Vx>"
  From/1 -> MATLAB Function16/1(Fx_fl)
  From5/1 -> MATLAB Function16/2(Fy_fl)
  From6/1 -> MATLAB Function16/3(Sx_fl)
  From7/1 -> MATLAB Function16/4(Sy_fl)
  Constant30/1 -> MATLAB Function16/9(lf)
  Constant78/1 -> MATLAB Function16/10(twf)
  Constant92/1 -> MATLAB Function22/10(twf)
  Constant90/1 -> MATLAB Function22/9(lf)
  From41/1 -> MATLAB Function22/4(Sy_fr)
  From40/1 -> MATLAB Function22/3(Sx_fr)
  From36/1 -> MATLAB Function22/2(Fy_fr)
  From8/1 -> MATLAB Function22/1(Fx_fr)
  Bus Selector19/1 -> MATLAB Function22/5(Vx)  "<Vx>"
  Bus Selector19/2 -> MATLAB Function22/6(Vy)  "<Vy>"
  Bus Selector19/3 -> MATLAB Function22/7(r)  "<r_d>"
  Bus Selector19/4 -> MATLAB Function22/8(delta_f)  "<detal_f>"
  MATLAB Function16/1(Px_fl) -> Scope10/1
  MATLAB Function16/2(Py_fl) -> Scope10/2
  MATLAB Function22/1(Px_fr) -> Scope11/1
  MATLAB Function22/2(Py_fr) -> Scope11/2
  MATLAB Function24/2(Py_rl) -> Scope12/2
  MATLAB Function24/1(Px_rl) -> Scope12/1
  Bus Selector20/3 -> MATLAB Function24/7(r)  "<r_d>"
  Bus Selector20/2 -> MATLAB Function24/6(Vy)  "<Vy>"
  Bus Selector20/1 -> MATLAB Function24/5(Vx)  "<Vx>"
  From45/1 -> MATLAB Function24/1(Fx_rl)
  From42/1 -> MATLAB Function24/2(Fy_rl)
  From43/1 -> MATLAB Function24/3(Sx_rl)
  From44/1 -> MATLAB Function24/4(Sy_rl)
  Constant94/1 -> MATLAB Function24/9(twr)
  Constant93/1 -> MATLAB Function24/8(lr)
  Constant95/1 -> MATLAB Function25/8(lr)
  Constant96/1 -> MATLAB Function25/9(twr)
  From48/1 -> MATLAB Function25/4(Sy_rr)
  From47/1 -> MATLAB Function25/3(Sx_rr)
  From46/1 -> MATLAB Function25/2(Fy_rr)
  From49/1 -> MATLAB Function25/1(Fx_rr)
  Bus Selector21/1 -> MATLAB Function25/5(Vx)  "<Vx>"
  Bus Selector21/2 -> MATLAB Function25/6(Vy)  "<Vy>"
  Bus Selector21/3 -> MATLAB Function25/7(r)  "<r_d>"
  MATLAB Function25/1(Px_rr) -> Scope13/1
  MATLAB Function25/2(Py_rr) -> Scope13/2
  [Fx_fl] -> Mux6/1
  [Fx_fr] -> Mux6/2
  [Fx_rl] -> Mux6/3
  [Fx_rr] -> Mux6/4
  Mux6/1 -> [Fx]
  Mux7/1 -> [Fy]
  [Fy_rr] -> Mux7/4
  [Fy_rl] -> Mux7/3
  [Fy_fr] -> Mux7/2
  [Fy_fl] -> Mux7/1
  [Vsx_fl] -> Mux8/1
  [Vsx_fr] -> Mux8/2
  [Vsy_rl] -> Mux8/3
  [Vsy_rr] -> Mux8/4
  Mux8/1 -> [Vsy]
  MATLAB Function5/3(Vsx_fr) -> [Vsx_fr]
  MATLAB Function5/4(Vsy_fr) -> [Vsy_fr]
  Mux9/1 -> [Vsx]
  [Vsx_rr] -> Mux9/4
  [Vsx_rl] -> Mux9/3
  [Vsx_fr] -> Mux9/2
  [Vsy_fl] -> Mux9/1
  MATLAB Function21/2(E_lat_J) -> Add1/2, Display4/1, Scope14/2
  MATLAB Function21/1(E_long_J) -> Scope14/1, Add1/1, Display6/1
  [Fx] -> MATLAB Function21/1(Fx)
  [Fy] -> MATLAB Function21/2(Fy)
  [Vsx] -> MATLAB Function21/3(Vsx)
  [Vsy] -> MATLAB Function21/4(Vsy)
  Constant97/1 -> MATLAB Function21/5(dt)
  Mux/1 -> [x_ref]
  MATLAB Function3/6(Debug_Info) -> Scope/2
  Bus Selector23/1 -> MATLAB Function17/2(delta_f)  "<detal_f>"
  Bus Selector6/3 -> 侧偏角计算/3(r)  "<r_d>"
  Bus Selector/11 -> Mu2/1, To Workspace13/1, Radius3/1, Mu13/1  "<Station>"
  Bus Selector22/1 -> Mu3/1, Mu14/1  "<Station>"
  Bus Selector23/2 -> Bus Selector22/1, Mu4/1  "<Station>"
  Bus Selector10/2 -> Mu5/1  "<Station>"
  Bus Selector12/2 -> Mu6/1  "<Station>"
  Bus Selector11/2 -> Mu7/1  "<Station>"
  Bus Selector13/2 -> Mu8/1  "<Station>"
  Bus Selector27/4 -> Mu9/1  "<Station>"
  Add1/1 -> Display5/1, Scope23/1
  Bus Selector6/2 -> 侧偏角计算/1(Vx)  "<Vx>"
  Bus Selector27/1 -> MATLAB Function19/1(Vx)  "<Vx>"
  Bus Selector24/1 -> Vx1/1  "<Station>"
  Bus Selector23/3 -> MATLAB Function17/1(Vx), Global_Target_Speed/1  "<Vx>"
  Bus Selector15/2 -> Scope8/1, Vx2/1, MU/1, Radius1/1, Add5/2  "<Station>"
  MU/1 -> MATLAB Function14/3(Mu_current), MATLAB Function23/11(Mu_Current), To Workspace14/1  "Mu_now"
  Add5/1 -> Mu12/1, Radius2/1
  Gain2/1 -> Add5/1
  Mu12/1 -> MATLAB Function14/5(Mu_preview)  "Mu_fut"
  Radius2/1 -> MATLAB Function14/6(Kappa_preview)  "Curv_fut"
  Mu13/1 -> MATLAB Function/9(Mu_in)
  Mu14/1 -> MATLAB Function15/12(Mu_in)
  Gain/1 -> Scope22/1, Gain2/1, Scope21/1, MATLAB Function14/1(Vx_kmh)
  Radius3/1 -> MATLAB Function/10(Curv_in)  "Curv_prev"
  Bus Selector16/1 -> MATLAB Function/11(Delta_f_in)  "<detal_f>"
  Bus Selector26/2 -> MATLAB Function15/11(delta_steering)  "<detal_f>"
  MATLAB Function14/1(NN_Weights) -> MATLAB Function/6(NN_Weights), Scope19/1, To Workspace2/1
  Bus Selector7/2 -> MATLAB Function5/1(Vx)  "<Vx>"
  Bus Selector5/2 -> unitire轮胎力/1(Vx)  "<Vx>"
  Bus Selector8/2 -> MATLAB Function6/1(Vx)  "<Vx>"
  Bus Selector9/2 -> MATLAB Function7/1(Vx)  "<Vx>"
  Bus Selector1/1 -> Bus Creator/1  "<Vx>"
  Bus Selector1/2 -> Bus Creator/2  "<detal_f>"
  Vx1/1 -> MATLAB Function18/1(Vx_target_input)
  Bus Selector26/1 -> Scope37/2, MATLAB Function15/2(Vx_act_raw)  "<Vx>"
  [SI] -> MATLAB Function15/15(SI_in)
  Bus Selector26/3 -> MATLAB Function15/14(Beta_in), Radius4/1  "<Beta>"
  Radius4/1 -> MATLAB Function15/13(Curv_in)  "Curv_prev"
  Bus Selector27/2 -> MATLAB Function19/2(Beta)  "<Beta>"
  Radius1/1 -> MATLAB Function14/4(Kappa_current)  "Curv_now"
  Bus Selector15/1 -> Gain/1  "<Vx>"
  Vx2/1 -> MATLAB Function14/2(Vref_kmh)
  Bus Selector23/4 -> Scope30/4  "<r_d>"
  [T_ref_upper] -> MATLAB Function12/2(T_sum_ref)
  Constant61/1 -> MATLAB Function12/3(dt)
  [T_ZY_FL] -> Mux3/1
  [T_ZY_FR] -> Mux3/2
  [T_ZY_RL] -> Mux3/3
  [T_ZY_RR] -> Mux3/4
  Mux3/1 -> [T_sum_out]
  [T_sum_out] -> MATLAB Function12/1(T_sum_out)
  MATLAB Function12/1(eT) -> Scope27/1
  MATLAB Function12/2(eT_percent) -> Scope27/2
  MATLAB Function12/3(I_err) -> Scope29/1
  MATLAB Function12/4(I_ref) -> Scope29/2
  MATLAB Function12/5(T_sum_err) -> Scope29/3
  Step/1 -> MATLAB Function12/4(is_reset)
  [Sx_fl] -> Mux10/1
  [Sx_fr] -> Mux10/2
  [Sy_rl] -> Mux10/3
  [Sx_rr] -> Mux10/4
  Mux10/1 -> [Sx_vec]
  [Sx_vec] -> MATLAB Function26/1(Sx_vec)
  [Fx] -> MATLAB Function26/2(Fx_vec)
  [Fy] -> MATLAB Function26/3(Fy_vec)
  Bus Selector18/1 -> Mux12/1  "<Fz11>"
  Bus Selector18/2 -> Mux12/2  "<Fz12>"
  Bus Selector18/3 -> Mux12/3  "<Fz21>"
  Bus Selector18/4 -> Mux12/4  "<Fz22>"
  Mux12/1 -> MATLAB Function26/4(Fz_vec)
  MATLAB Function26/1(Sx_abs_vec) -> To Workspace17/1
  MATLAB Function26/2(Sx_max) -> To Workspace18/1
  MATLAB Function26/3(Sx_rms) -> [Sx_rms], To Workspace19/1
  MATLAB Function26/4(Eta_vec) -> To Workspace20/1
  MATLAB Function26/5(Eta_max) -> To Workspace21/1
  MATLAB Function26/6(Eta_rms) -> To Workspace22/1
  MATLAB Function26/7(Debug_Info) -> To Workspace23/1
  [Sx_rms] -> MATLAB Function27/1(Sx_rms)
  MATLAB Function27/1(I_Sx) -> Display8/1, To Workspace24/1
  MATLAB Function27/2(I_Sx_norm) -> To Workspace25/1
  MATLAB Function27/3(I_Debug) -> To Workspace26/1
  Constant75/1 -> Mux13/1
  Constant76/1 -> Mux13/2
  Constant83/1 -> Mux13/3
  Constant85/1 -> Mux13/4
  Constant87/1 -> Mux13/5

== matlab function PGA_MPC_MODEL/Subsystem1/MATLAB Function3 ==
  data: T_total_req input; T_ref_fl output; w_fl input; w_fr input; w_rl input; w_rr input; Fz_fl input; T_ref_fr output; Fz_fr input; Fz_rl input; Fz_rr input; Ay_in input; SI_in input; Mu_in input; Lat_Error_in input; MotorData parameter; T_motor_max input; T_ref_rl output; T_ref_rr output; Mode_Out output; dt input; Debug_Info output
function [T_ref_fl, T_ref_fr, T_ref_rl, T_ref_rr, Mode_Out, Debug_Info] = ...
Upper_Layer_Optimization_Based(T_total_req, w_fl, w_fr, w_rl, w_rr, ...
Fz_fl, Fz_fr, Fz_rl, Fz_rr, ...
Ay_in, SI_in, Mu_in, Lat_Error_in, ... 
MotorData, T_motor_max, dt)
%#codegen
% =========================================================================
% 上层控制器 v5.0 (自适应抗“画龙”平稳版
% 
% [核心突破]
% 1. 引入 Risk_Smooth 历史低通滤波，并平滑 Sigmoid 函数，彻底治愈模式切换的神经质跳变。
% 2. 引入动态模式切换惩罚 (W_switch_dyn)：路越滑(Mu越小)，越不准随便切换驱动模式，锁死稳定分配。
% =========================================================================
%% 1. 初始化与数据加载
persistent last_lambda 
persistent map_x_vec map_y_vec map_z_mat 
persistent T_req_smooth Risk_Smooth
coder.varsize('map_x_vec', [1, 5000], [0, 1]); 
coder.varsize('map_y_vec', [1, 5000], [0, 1]);
coder.varsize('map_z_mat', [5000, 5000], [1, 1]);

if isempty(last_lambda)
last_lambda = 0.5; % 默认四驱起步
T_req_smooth = 0;
Risk_Smooth = 0.0; % 初始化风险滤波状态
raw_x = [0, 100, 200]; 
raw_y = [0, 100, 200]; 
raw_z = 0.9 * ones(3,3);
if ~isempty(MotorData)
if isfield(MotorData, 'Speed_Axis'), raw_x = double(MotorData.Speed_Axis); end
if isfield(MotorData, 'Torque_Axis'), raw_y = double(MotorData.Torque_Axis); end
if isfield(MotorData, 'Eff_Map'), raw_z = double(MotorData.Eff_Map); end
end
map_x_vec = reshape(raw_x, 1, []); 
map_y_vec = reshape(raw_y, 1, []); 
[nr, nc] = size(raw_z);
len_x = length(map_x_vec); 
len_y = length(map_y_vec); 
if nr == len_x && nc == len_y
map_z_mat = raw_z';
elseif nr == len_y && nc == len_x
map_z_mat = raw_z;
else
map_z_mat = raw_z; 
end
end

%% 2. 信号预处理
Raw_T_req = double(T_total_req(1));
T_req_smooth = 0.9 * T_req_smooth + 0.1 * Raw_T_req;
T_req = T_req_smooth;
T_lim = double(T_motor_max(1));

% 获取当前路面附着系数
Mu = max(0.15, double(Mu_in(1))); 

w_vec = [double(w_fl), double(w_fr), double(w_rl), double(w_rr)];
w_avg_rpm = (mean(abs(w_vec)) + 1e-3); 
w_query = w_avg_rpm; 
Fz_F_Tot = double(Fz_fl + Fz_fr) + 1.0;
Fz_R_Tot = double(Fz_rl + Fz_rr) + 1.0;

%% 3. ★ 风险评估 (动态平滑版：彻底解决画龙跳变) ★
Ay_val = abs(double(Ay_in(1)));
Ay_Max = Mu * 9.81; 
R_Ay = max(0, (Ay_val / (Ay_Max + 0.1)) - 0.7) / 0.3; 
SI_val = double(SI_in(1));
R_SI = clamp((SI_val - 0.5) / 0.4, 0, 1);
Lat_val = abs(double(Lat_Error_in(1)));
R_Lat = clamp((Lat_val - 0.5) / 0.5, 0, 1);

Raw_Risk = max([R_Ay, R_SI, R_Lat]);

% 核心1：引入一阶低通滤波，抚平突发峰值，让风险感知变得稳重
Risk_Smooth = 0.90 * Risk_Smooth + 0.10 * Raw_Risk;

% 核心2：使用平缓的 Sigmoid (-10 代替 -20)，消除非黑即白的神经质跳变
% 保证在危险时(Risk_Smooth>0.8)依然能逼近 1.0 锁定四驱。
Risk_Factor = 1 / (1 + exp(-10.0 * (Risk_Smooth - 0.5)));
Risk_Factor = clamp(Risk_Factor, 0, 1);

%% 4. 可行域收缩 (危险时强制回退四驱)
if T_req >= 0
l_min_phys = max(0, 1 - (2*T_lim / (T_req + 1e-6)));
l_max_phys = min(1, (2*T_lim / (T_req + 1e-6)));
else
l_min_phys = max(0, 1 - (2*T_lim / (abs(T_req) + 1e-6)));
l_max_phys = min(1, (2*T_lim / (abs(T_req) + 1e-6)));
end
l_min_safe = 0.0 + 0.5 * Risk_Factor;
l_max_safe = 1.0 - 0.5 * Risk_Factor;
l_start = max(l_min_phys, l_min_safe);
l_end = min(l_max_phys, l_max_safe);
if l_start > l_end, l_start = 0.5; l_end = 0.5; end

%% 5. 物理感知代价函数优化 (★ 动态路面锁定版 ★)
num_grid = 21; 
step_val = (l_end - l_start) / (num_grid - 1);
min_cost = 1e12; 
best_lambda = last_lambda; 

% 核心3：动态切换惩罚。
% 柏油路(Mu=0.85)时惩罚约为210，允许灵活切换追求经济性；
% 冰面(Mu=0.30)时惩罚飙升至500，死死锁住当前最优分配，坚决不准切换导致打滑！
W_switch_dyn = 200.0 * (1.0 / (Mu + 0.1)); 

W_tire_loss = 2.0; 

for i = 0 : num_grid-1
curr_lambda = l_start + i * step_val;
T_f = T_req * curr_lambda;
T_r = T_req * (1 - curr_lambda);
P_loss_motor_f = calc_power_loss(T_f/2, w_query, map_x_vec, map_y_vec, map_z_mat) * 2;
P_loss_motor_r = calc_power_loss(T_r/2, w_query, map_x_vec, map_y_vec, map_z_mat) * 2;
P_tire_f = W_tire_loss * (T_f^2) / (Fz_F_Tot);
P_tire_r = W_tire_loss * (T_r^2) / (Fz_R_Tot);
J_energy = P_loss_motor_f + P_loss_motor_r + P_tire_f + P_tire_r;
% 应用动态抗震荡切换惩罚
J_switch = W_switch_dyn * (curr_lambda - last_lambda)^2; 
Total_Cost = J_energy + J_switch;
if Total_Cost < min_cost
min_cost = Total_Cost;
best_lambda = curr_lambda;
end
end

% 极致滤波，锁定最终指令
lambda_smooth = 0.95 * last_lambda + 0.05 * best_lambda;
lambda_smooth = clamp(lambda_smooth, l_start, l_end);
last_lambda = lambda_smooth;

%% 6. 输出分配 (按载荷稳态预分配)
Front_Tot = T_req * lambda_smooth;
Rear_Tot = T_req * (1 - lambda_smooth);
Fz_F_Tot = Fz_fl + Fz_fr + 1;
Fz_R_Tot = Fz_rl + Fz_rr + 1;

T_ref_fl = Front_Tot * (Fz_fl / Fz_F_Tot);
T_ref_fr = Front_Tot * (Fz_fr / Fz_F_Tot);
T_ref_rl = Rear_Tot * (Fz_rl / Fz_R_Tot);
T_ref_rr = Rear_Tot * (Fz_rr / Fz_R_Tot);

Mode_Out = 1.0 - lambda_smooth; 
Debug_Info = [lambda_smooth; min_cost; Risk_Factor; Raw_Risk; W_switch_dyn];
end

%% === 辅助函数：查表与损耗计算 ===
function P_loss = calc_power_loss(T_val, w_val, x_axis, y_axis, z_map)
T_abs = abs(T_val); 
w_abs = abs(w_val);
if T_abs < 0.1, P_loss = 0; return; end
eff = manual_bilinear_interp(x_axis, y_axis, z_map, w_abs, T_abs);
eff = max(min(eff, 0.98), 0.05); 
P_mech = T_abs * w_abs; 
P_loss = P_mech * (1.0/eff - 1.0);
end

function val = manual_bilinear_interp(X, Y, Z, xq, yq)
xq = max(min(xq, X(end)), X(1)); 
yq = max(min(yq, Y(end)), Y(1));
idx_x = 1; 
for k = 1:length(X)-1
if xq >= X(k) && xq <= X(k+1), idx_x = k; break; end
end
if idx_x >= length(X), idx_x = length(X)-1; end
idx_y = 1; 
for k = 1:length(Y)-1
if yq >= Y(k) && yq <= Y(k+1), idx_y = k; break; end
end
if idx_y >= length(Y), idx_y = length(Y)-1; end
u = (xq - X(idx_x)) / (X(idx_x+1) - X(idx_x) + 1e-9);
v = (yq - Y(idx_y)) / (Y(idx_y+1) - Y(idx_y) + 1e-9);
val = (1-v) * ((1-u)*Z(idx_y, idx_x) + u*Z(idx_y, idx_x+1)) + ...
v * ((1-u)*Z(idx_y+1, idx_x) + u*Z(idx_y+1, idx_x+1));
end

function y = clamp(x, lo, hi), y = max(min(x, hi), lo); end

== matlab function PGA_MPC_MODEL/Subsystem1/MATLAB Function4 ==
  data: Vx input; beta_ref output; delta_f input; lf input; lr input; Kyf input; Kyr input; m input; dt input
function beta_ref = Beta_Ref_Generation_Constant(Vx, delta_f, lf, lr, Kyf, Kyr, m, dt)
% =========================================================================
% 质心侧偏角参考值生成 (终极数学修正版)
% 修复：原公式量纲错误，现替换为严谨的 2DOF 稳态响应物理公式
% =========================================================================
    % 1. 输入预处理
    Vx_safe = max(abs(Vx), 1.0) * sign(Vx); % 避免低速奇异
    L = lf + lr;

    % 2. 转换为整轴侧偏刚度 (极度重要)
    Kyf_axle = Kyf * 2; 
    Kyr_axle = Kyr * 2;

    % 3. 计算稳态横摆增益 Ks 
    % 注意：因为已经用了整轴刚度，公式分母是 L^2 而不是 2L^2
    K_s = (m / L^2) * (lr / Kyf_axle - lf / Kyr_axle);

    % 4. 使用正确的稳态质心侧偏角公式
    % 公式: beta = delta * (lr - lf*m*Vx^2 / (Kyr_axle*L)) / (L * (1 + Ks*Vx^2))
    term_num = lr - (lf * m * Vx_safe^2) / (Kyr_axle * L);
    term_den = L * (1 + K_s * Vx_safe^2);
    
    beta_ref_raw = (term_num / term_den) * delta_f;

    % 5. 低通滤波 (模拟真实车辆惯性延迟，必须保留！)
    persistent beta_prev;
    if isempty(beta_prev)
        beta_prev = 0;
    end
    tau = 0.05;
    beta_smoothed = (dt * beta_ref_raw + tau * beta_prev) / (tau + dt);

    % 6. 幅值限制
    beta_max = 8 * pi / 180;
    beta_ref = max(min(beta_smoothed, beta_max), -beta_max);

    % 更新历史值
    beta_prev = beta_ref;
    beta_ref = real(beta_ref);
end

== matlab function PGA_MPC_MODEL/Subsystem1/MATLAB Function2 ==
  settings: updateMethod=DISCRETE
  data: T_fl input; P_total_kW output; T_fr input; T_rl input; T_rr input; w_fl input; w_fr input; w_rl input; w_rr input; Map_Spd input; Map_Trq input; Map_Eff input; dt input; is_reset input; E_total_kWh output; P_avg_kW output
function [P_total_kW, E_total_kWh, P_avg_kW] = Calc_Energy_Internal_Map(...
    T_fl, T_fr, T_rl, T_rr, ...       
    w_fl, w_fr, w_rl, w_rr, ...       
    Map_Spd, Map_Trq, Map_Eff, ...    
    dt, is_reset)                     
%#codegen
% =========================================================================
% 全工况能耗计算器 v11.1 (最终版)
% [核心特性]
% 1. 完整覆盖驱动与制动回收双象限查表 (原样保留负转矩传入查表)。
% 2. 包含 35% 低扭效率兜底机制，避免除零或无穷大功率奇点，更贴合实际物理下限。
% 3. 包含车规级制动回收保护：低速 (<5 rad/s) 与低效 (<20%) 区间强制切断。
% =========================================================================
    persistent E_accumulated_J Total_Time_s
    if isempty(E_accumulated_J) || is_reset
        E_accumulated_J = 0;
        Total_Time_s = 0;
    end
    
    T_vec = [double(T_fl), double(T_fr), double(T_rl), double(T_rr)];
    w_vec = [double(w_fl), double(w_fr), double(w_rl), double(w_rr)];
    
    % --- ★ 轮毂电机物理与工程参数 ★ ---
    i_gear = 1.0; % 直驱轮毂电机减速比
    P_base_loss_W = 150.0; % 逆变器与控制器的基础待机损耗 (W)
    
    vec_x_rad = double(Map_Spd); 
    vec_y_nm  = double(Map_Trq); 
    mat_eff   = double(Map_Eff)';
    
    P_elec_W_vec = zeros(1, 4);
    
    for i = 1:4
        T_wheel = T_vec(i);     
        w_wheel_rads = w_vec(i);     
        
        % 1. 计算电机端工况
        % ★ 核心：速度取绝对值，扭矩保留正负号，以精确匹配四象限 Map 表！
        T_motor = T_wheel / i_gear; 
        w_motor_rads = abs(w_wheel_rads) * i_gear; 
        
        % 计算轮端机械功率 (驱动时为正，制动反拖时为负)
        P_mech_wheel = T_wheel * w_wheel_rads; 
        
        % 2. 极端静止/空转工况拦截
        if abs(w_wheel_rads) < 1.0
            % 车辆基本停稳，电机停止输出，彻底切断电能消耗
            P_elec = 0; 
        elseif abs(T_wheel) < 3.0 
            % 车辆滑行或该轮被上层分配 0 扭矩，仅消耗基础待机电量
            P_elec = P_base_loss_W; 
        else
            % 3. 正常工况：查表获取当前效率
            eff_raw = manual_interp2(vec_x_rad, vec_y_nm, mat_eff, w_motor_rads, T_motor);
            
            % 4. 驱动与制动能量流向计算
            if P_mech_wheel > 0
                % =========================================================
                % 【驱动耗电模式】
                % 引入 35% 的工程效率兜底，防止极低扭矩时的能耗被数学奇点无限放大
                % 消耗电功率 = (机械功率 / 效率) + 基础待机功耗
                % =========================================================
                eff_final = max(eff_raw, 0.35); 
                P_elec = (P_mech_wheel / eff_final) + P_base_loss_W;
                
            else
                % =========================================================
                % 【制动回收模式 (Regenerative Braking)】
                % P_mech_wheel 为负值
                % =========================================================
                if eff_raw < 0.20 || w_motor_rads < 5.0 
                    % 工程保护机制：低速域或极低效率域，强行切断激磁回收
                    % 避免开关损耗大于回收收益的现象
                    P_elec = P_base_loss_W; 
                else
                    % 物理能量守恒：
                    % 负的机械功率 * 效率 = 缩水的负电功率 (代表实际回充至母线的电量)
                    % 加上正的待机功耗，进一步减少了最终充入电池的能量
                    P_elec = (P_mech_wheel * eff_raw) + P_base_loss_W; 
                end
            end
        end
        % 记录单个车轮的总电功率
        P_elec_W_vec(i) = P_elec;
    end
    
    % --- 5. 整车能耗累加与统计 ---
    P_total_W = sum(P_elec_W_vec);       % 整车瞬时总功率 (W)
    P_total_kW = P_total_W / 1000;       % 整车瞬时总功率 (kW)
    
    % 焦耳积分 (J = W * s)
    E_accumulated_J = E_accumulated_J + P_total_W * double(dt);
    Total_Time_s = Total_Time_s + double(dt);
    
    % 转换为 kWh (1 kWh = 3.6e6 J)
    E_total_kWh = E_accumulated_J / 3.6e6;
    
    % 计算全历程平均功率
    if Total_Time_s > 1e-3
        P_avg_kW = (E_accumulated_J / Total_Time_s) / 1000;
    else
        P_avg_kW = 0;
    end
end

% ==== 手写双线性插值函数 (Bilinear Interpolation) ====
function val = manual_interp2(X, Y, Z, xq, yq)
    % 边界钳位保护
    xq_c = max(min(xq, X(end)), X(1));
    yq_c = max(min(yq, Y(end)), Y(1));
    
    % 寻找 X 轴索引
    idx_x = 1;
    for k = 1:length(X)-1
        if xq_c >= X(k) && xq_c <= X(k+1), idx_x = k; break; end
    end
    
    % 寻找 Y 轴索引
    idx_y = 1;
    for k = 1:length(Y)-1
        if yq_c >= Y(k) && yq_c <= Y(k+1), idx_y = k; break; end
    end
    
    x1 = X(idx_x); x2 = X(idx_x+1);
    y1 = Y(idx_y); y2 = Y(idx_y+1);
    
    % 归一化局部坐标
    if abs(x2-x1)<1e-9, u=0; else, u=(xq_c-x1)/(x2-x1); end
    if abs(y2-y1)<1e-9, v=0; else, v=(yq_c-y1)/(y2-y1); end
    
    % 四点提取
    f11 = Z(idx_y,   idx_x);
    f21 = Z(idx_y,   idx_x+1);
    f12 = Z(idx_y+1, idx_x);
    f22 = Z(idx_y+1, idx_x+1);
    
    % 双线性加权
    val = (1-v)*((1-u)*f11 + u*f21) + v*((1-u)*f12 + u*f22);
    
    if isnan(val), val = 0.01; end
end

== matlab function PGA_MPC_MODEL/Subsystem1/MATLAB Function12 ==
  data: T_sum_out input; eT output; T_sum_ref input; dt input; is_reset input; eT_percent output; I_err output; I_ref output; T_sum_err output
function [eT, eT_percent, I_err, I_ref, T_sum_err] = Calc_Torque_Tracking_Error( ...
    T_sum_out, T_sum_ref, dt, is_reset)
%#codegen
% =========================================================================
% Total Torque Tracking Error Index
%
% eT = integral(|T_sum_out - T_sum_ref| dt) / integral(|T_sum_ref| dt)
%
% 用途：
% 1) 判断下层 MPC 是否过度偏离上层总需求转矩
% 2) 解释 W_sum 降低后是否只是靠“少给转矩”换来低能耗和高稳定性
% =========================================================================

    persistent I_err_acc I_ref_acc

    if isempty(I_err_acc) || double(is_reset(1)) > 0.5
        I_err_acc = 0.0;
        I_ref_acc = 0.0;
    end

    dt_in = double(dt(1));
    if isnan(dt_in) || isinf(dt_in) || dt_in <= 1e-6
        dt_in = 0.01;
    end

    T_out = double(T_sum_out(1));
    T_ref = double(T_sum_ref(1));

    if isnan(T_out) || isinf(T_out)
        T_out = 0.0;
    end

    if isnan(T_ref) || isinf(T_ref)
        T_ref = 0.0;
    end

    T_sum_err = T_out - T_ref;

    I_err_acc = I_err_acc + abs(T_sum_err) * dt_in;
    I_ref_acc = I_ref_acc + abs(T_ref) * dt_in;

    I_err = I_err_acc;
    I_ref = I_ref_acc;

    if I_ref_acc > 1e-6
        eT = I_err_acc / I_ref_acc;
    else
        eT = 0.0;
    end

    eT_percent = 100.0 * eT;
end
